simulink model "SCCS_Integrated_Test_03"  (R2024a)
settings: Solver=ode3  StartTime=0.0  StopTime=15  FixedStep=0.01  RelTol=1e-3
settings Model: Creator=Kishore  LastModifiedBy=Kishore

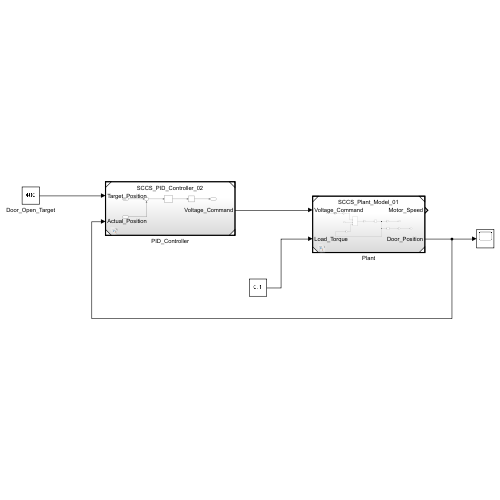
[thumbnail: Simulink's stored preview of the top-level diagram]
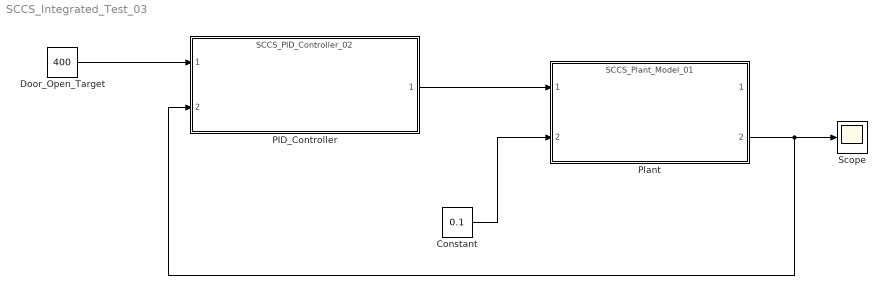
== system SCCS_Integrated_Test_03 ==
  Constant : Constant  Value=0.1
  Door_Open_Target : Constant  Value=400
  PID_Controller : ModelReference  ModelNameDialog=SCCS_PID_Controller_02.slx  SimulationMode=Normal  ModelReferenceVersion=1.13
  Plant : ModelReference  ModelNameDialog=SCCS_Plant_Model_01.slx  SimulationMode=Normal  ModelReferenceVersion=1.15
  Scope : Scope
  wires:
  Door_Open_Target/1 -> PID_Controller/1
  PID_Controller/1 -> Plant/1
  Plant/2 -> PID_Controller/2, Scope/1
  Constant/1 -> Plant/2
